simulink model "water"  (R2017b)
settings: Solver=VariableStepAuto  StartTime=0.0  StopTime=100  RelTol=1e-3
libraries: fuzblock x1, simulink x1
settings Model: Creator=Silicon  LastModifiedBy=Silicon

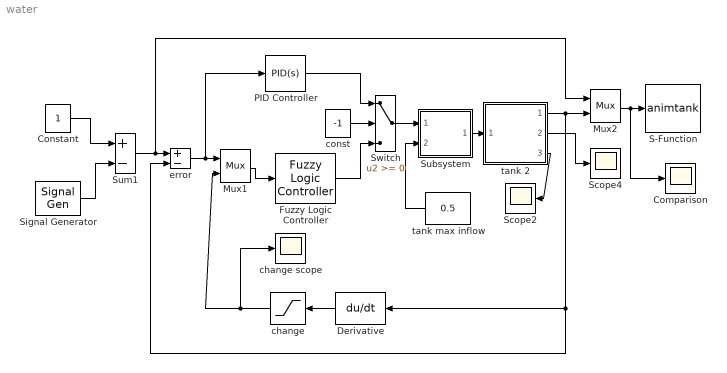
== system water ==
  Comparison : Scope
  Constant : Constant
  Derivative : Derivative
  Fuzzy Logic Controller : fuzblock/Fuzzy Logic  Controller  FIS='tank2.fis'  OutputSampleNumber=101  DataType=double  FuzzifiedInputs=off  RuleFiringStrengths=off  RuleOutputs=off  AggregatedOutputs=off  SimulateUsing=Interpreted execution
  Mux1 : Mux  Inputs=2
  Mux2 : Mux  Inputs=2
  PID Controller : simulink/Continuous/PID Controller  Controller=PID  TimeDomain=Continuous-time  SampleTime=-1  IntegratorMethod=Forward Euler  FilterMethod=Forward Euler  Form=Parallel  UseFilter=on  ControllerParametersSource=internal  P=2  I=0  D=1  N=100  InitialConditionSource=internal  InitialConditionForIntegrator=0  InitialConditionForFilter=0  ExternalReset=none  LimitOutput=off  UpperSaturationLimit=inf  LowerSaturationLimit=-inf  LinearizeAsGain=off  AntiWindupMode=none  Kb=1  TrackingMode=off  Kt=1  PParamMin=[]  PParamMax=[]  IParamMin=[]  IParamMax=[]  DParamMin=[]  DParamMax=[]  NParamMin=[]  NParamMax=[]  KbParamMin=[]  KbParamMax=[]  KtParamMin=[]  KtParamMax=[]  POutMin=[]  POutMax=[]  IOutMin=[]  IOutMax=[]  DOutMin=[]  DOutMax=[]  NOutMin=[]  NOutMax=[]  KbOutMin=[]  KbOutMax=[]  KtOutMin=[]  KtOutMax=[]  IntegratorOutMin=[]  IntegratorOutMax=[]  FilterOutMin=[]  FilterOutMax=[]  SumOutMin=[]  SumOutMax=[]  SumI1OutMin=[]  SumI1OutMax=[]  SumI2OutMin=[]  SumI2OutMax=[]  SumI3OutMin=[]  SumI3OutMax=[]  SumDOutMin=[]  SumDOutMax=[]  SaturationOutMin=[]  SaturationOutMax=[]  IntegratorContinuousStateAttributes=''  IntegratorStateMustResolveToSignalObject=off  IntegratorRTWStateStorageClass=Auto  FilterContinuousStateAttributes=''  FilterStateMustResolveToSignalObject=off  FilterRTWStateStorageClass=Auto  DifferentiatorICPrevScaledInput=0  DifferentiatorOutMin=[]  DifferentiatorOutMax=[]  InitialConditionSetting=State (most efficient)  FilterDiffOutCoefMin=[]  FilterDiffOutCoefMax=[]  SumDenOutMin=[]  SumDenOutMax=[]  SumNumOutMin=[]  SumNumOutMax=[]  ReciprocalOutMin=[]  ReciprocalOutMax=[]  DivideOutMin=[]  DivideOutMax=[]  TunerSelectOption=Transfer Function Based (PID Tuner App)
  S-Function : S-Function  FunctionName=animtank  Parameters=1  SFunctionDeploymentMode=off  EnableBusSupport=off
  Scope2 : Scope
  Scope4 : Scope
  Signal Generator : SignalGenerator  WaveForm=square  Amplitude=0.500000  Frequency=0.100000  Units=rad/sec
  Subsystem : Subsystem  mask(Valve){InitialPosition=0}
      mask prompts: InitialPosition "Initial position [0=closed 1=open]:"
      mask help: Valve
      mask Display: disp('VALVE')
  Sum1 : Sum  Inputs=+-  SaturateOnIntegerOverflow=on  InputSameDT=on  OutDataTypeStr=Inherit: Same as first input
  Switch : Switch  SaturateOnIntegerOverflow=on  InputSameDT=on
  change : Saturate  UpperLimit=0.1  LowerLimit=-0.1
  change scope : Scope
  const : Constant  Value=-1
  error : Sum  Inputs=+-  SaturateOnIntegerOverflow=on  InputSameDT=on  OutDataTypeStr=Inherit: Same as first input
  tank 2 : Subsystem  mask(Water tank){ht=2, area=1, outletArea=0.05, overflowLimit=0, initialHt=0.5}
      mask prompts: ht "Height of tank (m):"; area "Bottom area (m^2):"; outletArea "Out pipe crossection (m^2):"; overflowLimit "Overflow sensor distance from top (m):"; initialHt "Initial level height (m):"
      mask help: Cylindrical water tank with overflow signal
      mask Display: disp('WATER\nTANK')
  tank max inflow : Constant  Value=0.5
  wires:
  const/1 -> Switch/2
  Mux1/1 -> Fuzzy Logic Controller/1
  PID Controller/1 -> Switch/1
  Fuzzy Logic Controller/1 -> Switch/3
  Mux2/1 -> S-Function/1, Comparison/1
  Signal Generator/1 -> Sum1/2
  Constant/1 -> Sum1/1
  change/1 -> Mux1/2, change scope/1
  Sum1/1 -> error/1, Mux2/1
  Subsystem/1(out flow) -> tank 2/1(flow in)
  Switch/1 -> Subsystem/1(control)
  Derivative/1 -> change/1
  tank 2/3(overflow flag) -> Scope2/1
  tank max inflow/1 -> Subsystem/2(source flow)
  tank 2/2(flow out) -> Scope4/1
  tank 2/1(water level) -> Mux2/2, error/2, Derivative/1
  error/1 -> Mux1/1, PID Controller/1

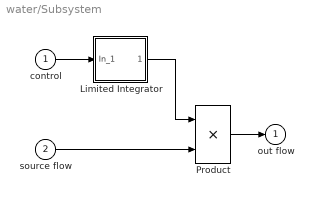
== system water/Subsystem ==
  control : Inport
  source flow : Inport  Port=2
  Limited Integrator : Subsystem  mask(Limited integrator.){lb=0, ub=1, xi=InitialPosition}
      mask prompts: lb "Lower bound:"; ub "Upper bound:"; xi "Initial condition"
      mask help: Limited integrator
      mask Help: Implements a limited integrator with \nan expression of the form:\n\nif(x<=lb and u<0) or (x>=ub and u>0)\n\txdot=0\nelse\n\txdot=u.
      mask Display: plot(-1,-0.2,3.5,1.2,[0.05,1,2,2.9],[0,0,1,1]);disp(' 1/s    ')
  Product : Product  SaturateOnIntegerOverflow=on  RndMeth=Zero  InputSameDT=on  OutDataTypeStr=Inherit: Same as first input
  out flow : Outport  InitialOutput=0
  wires:
  source flow/1 -> Product/2
  Product/1 -> out flow/1
  control/1 -> Limited Integrator/1(In_1)
  Limited Integrator/1(Out_1) -> Product/1

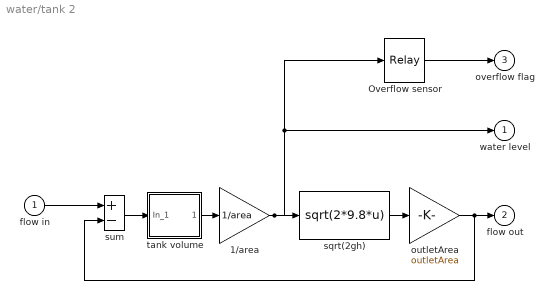
== system water/tank 2 ==
  flow in : Inport
  1/area : Gain  Gain=1/area  SaturateOnIntegerOverflow=on  OutDataTypeStr=Inherit: Same as input  ParamDataTypeStr=Inherit: Same as input
  Overflow sensor : Relay  OnSwitchValue=ht - overflowLimit  OffSwitchValue=ht - overflowLimit
  outletArea : Gain  Gain=outletArea  SaturateOnIntegerOverflow=on  OutDataTypeStr=Inherit: Same as input  ParamDataTypeStr=Inherit: Same as input
  sqrt(2gh) : Fcn  Expr=sqrt(2*9.8*u)
  sum : Sum  Inputs=+-  SaturateOnIntegerOverflow=on  InputSameDT=on  OutDataTypeStr=Inherit: Same as first input
  tank volume : Subsystem  mask(Limited integrator.){lb=0, ub=ht * area, xi=initialHt * area}
      mask prompts: lb "Lower bound:"; ub "Upper bound:"; xi "Initial condition"
      mask help: Limited integrator
      mask Help: Implements a limited integrator with \nan expression of the form:\n\nif(x<=lb and u<0) or (x>=ub and u>0)\n\txdot=0\nelse\n\txdot=u.
      mask Display: plot(-1,-0.2,3.5,1.2,[0.05,1,2,2.9],[0,0,1,1]);disp(' 1/s    ')
  water level : Outport  InitialOutput=0
  flow out : Outport  Port=2  InitialOutput=0
  overflow flag : Outport  Port=3  InitialOutput=0
  wires:
  outletArea/1 -> flow out/1, sum/2
  sqrt(2gh)/1 -> outletArea/1
  1/area/1 -> Overflow sensor/1, water level/1, sqrt(2gh)/1
  tank volume/1(Out_1) -> 1/area/1
  Overflow sensor/1 -> overflow flag/1
  flow in/1 -> sum/1
  sum/1 -> tank volume/1(In_1)

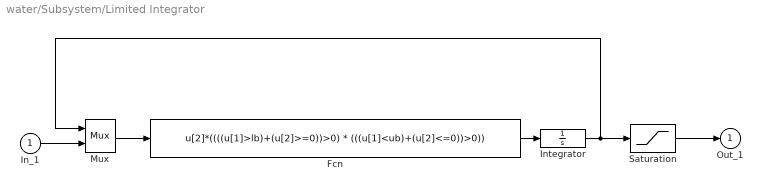
== system water/Subsystem/Limited Integrator ==
  In_1 : Inport
  Fcn : Fcn  Expr=u[2]*((((u[1]>lb)+(u[2]>=0))>0) * (((u[1]<ub)+(u[2]<=0))>0))
  Integrator : Integrator  InitialCondition=xi
  Mux : Mux  Inputs=2
  Saturation : Saturate  UpperLimit=ub  LowerLimit=lb
  Out_1 : Outport  InitialOutput=0
  wires:
  Integrator/1 -> Saturation/1, Mux/1
  Fcn/1 -> Integrator/1
  Mux/1 -> Fcn/1
  In_1/1 -> Mux/2
  Saturation/1 -> Out_1/1

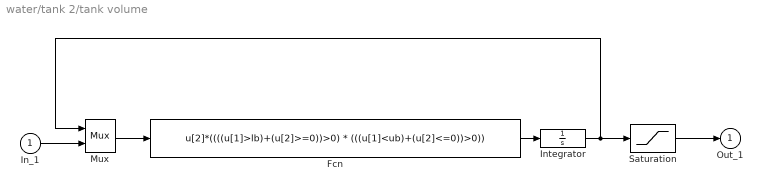
== system water/tank 2/tank volume ==
  In_1 : Inport
  Fcn : Fcn  Expr=u[2]*((((u[1]>lb)+(u[2]>=0))>0) * (((u[1]<ub)+(u[2]<=0))>0))
  Integrator : Integrator  InitialCondition=xi
  Mux : Mux  Inputs=2
  Saturation : Saturate  UpperLimit=ub  LowerLimit=lb
  Out_1 : Outport  InitialOutput=0
  wires:
  Integrator/1 -> Saturation/1, Mux/1
  Fcn/1 -> Integrator/1
  Mux/1 -> Fcn/1
  In_1/1 -> Mux/2
  Saturation/1 -> Out_1/1
